simulink library "adrc"  (Simulink 10.0)
settings: Solver=VariableStepAuto  StartTime=0.0  StopTime=10.0  RelTol=1e-3
undefined symbols (not defined in the file): DiscIntNeverNeededParam, Ts
libraries: fl_lib x7, nesl_utility x4, powerlib_meascontrol x1, eeGeneralControl x1
settings Model: Creator=Kamran  LastModifiedBy=Kamran

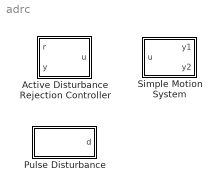
== system adrc ==
  Active Disturbance Rejection Controller : Subsystem  mask(Active Disturbance Rejection Controller){b=1, w=10, n=1, sat=inf}
      mask prompts: b "Input Gain (b)"; w "Bandwidth (w in rad/s)"; n "System Order"; sat "Output Saturation"
      mask help: This simulates a parametrized ADRC controller with minimal number of tuning parameters.
      mask init:
      | A = zeros(n + 1);
      | A(1:end-1, 2:end) = eye(n);
      | 
      | B = zeros(n + 1, 1);
      | B(end-1) = 1;
      | 
      | syms s;
      | 
      | eqn = (s + w) ^ n;
      | c = fliplr(sym2poly(eqn));
      | K = c(1:end-1);
      | 
      | eqn = (s + w) ^ (n + 1);
      | c = sym2poly(eqn);
      | L = c(2:end)';
      mask Display: disp("ADRC")
  Pulse Disturbance : Subsystem  mask{d=2.5, t=0.05, w=2, e=on}
      mask prompts: d "Transport Delay Time"; t "Disturbance Duration"; w "Amplitude"; e "Enabled"
      mask help: Simple pulse disturbance.
      mask Display: disp('Disturbance')
  Simple Motion System : Subsystem  mask{I=2, K=0.2, Taw=1e-3, Ts=1}
      mask prompts: I "Inertia"; K "Damping coefficient"; Taw "Drive Delay"; Ts "Sample Time"
      mask help: Simple motor motion control platform.
      mask Display: disp("Plant")

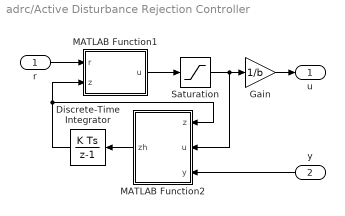
== system adrc/Active Disturbance Rejection Controller ==
  r : Inport
  y : Inport  Port=2
  Discrete-Time Integrator : DiscreteIntegrator  InitialCondition=zeros(1, n + 1)  SampleTime=-1  ICPrevOutput=DiscIntNeverNeededParam  ICPrevScaledInput=DiscIntNeverNeededParam
  Gain : Gain  Gain=1/b
  MATLAB Function1 : MATLAB Function  TreatAsAtomicUnit=on
  MATLAB Function2 : MATLAB Function  TreatAsAtomicUnit=on
  Saturation : Saturate  UpperLimit=sat*b  LowerLimit=-sat*b
  u : Outport  VectorParamsAs1DForOutWhenUnconnected=off
  wires:
  MATLAB Function1/1(u) -> Saturation/1
  r/1 -> MATLAB Function1/1(r)
  Saturation/1 -> Gain/1, MATLAB Function2/2(u)
  y/1 -> MATLAB Function2/3(y)
  Discrete-Time Integrator/1 -> MATLAB Function1/2(z), MATLAB Function2/1(z)
  MATLAB Function2/1(zh) -> Discrete-Time Integrator/1
  Gain/1 -> u/1

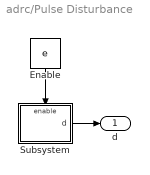
== system adrc/Pulse Disturbance ==
  Enable : Constant  Value=e  SampleTime=Ts
  Subsystem : Subsystem
  d : Outport  VectorParamsAs1DForOutWhenUnconnected=off
  wires:
  Enable/1 -> Subsystem/Enable
  Subsystem/1(d) -> d/1

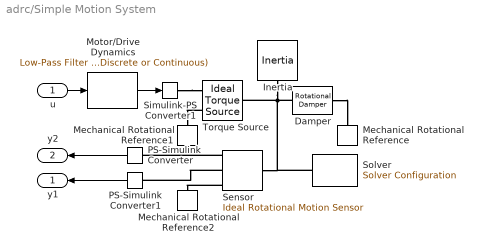
== system adrc/Simple Motion System ==
  u : Inport
  Damper : fl_lib/Mechanical/Rotational Elements/Rotational Damper  D=0.2 N*m/(rad/s)  w_specify=off  w_priority=None  w=0 rad/s  w_nominal_specify=off  w_nominal_unit=rad/s  w_nominal_value=1  t_specify=off  t_priority=None  t=0 N*m  t_nominal_specify=off  t_nominal_unit=N*m  t_nominal_value=1
  Inertia : fl_lib/Mechanical/Rotational Elements/Inertia  inertia=2 kg*m^2  w_specify=off  w_priority=High  w=0 rad/s  w_nominal_specify=off  w_nominal_unit=rad/s  w_nominal_value=1  t_specify=off  t_priority=None  t=0 N*m  t_nominal_specify=off  t_nominal_unit=N*m  t_nominal_value=1
  Mechanical Rotational Reference : fl_lib/Mechanical/Rotational Elements/Mechanical Rotational Reference
  Mechanical Rotational Reference1 : fl_lib/Mechanical/Rotational Elements/Mechanical Rotational Reference
  Mechanical Rotational Reference2 : fl_lib/Mechanical/Rotational Elements/Mechanical Rotational Reference
  Motor/Drive Dynamics : eeGeneralControl/Low-Pass Filter (Discrete or Continuous)  K=1  T=Taw  B=inf  A=-inf  Ts=-1  mask(Low-Pass Filter (Discrete or Continuous)){}
      settings: SourceProductName=Simscape Electrical
      mask Display:
      | % This is a new mask on top of the base mask.
      | % Use "View base mask" link below to see the base mask.
      | plot([0 1 2 3 4], [-1 -1 -2.5 -4 -4])
  PS-Simulink Converter : nesl_utility/PS-Simulink Converter  PhysicalDomain=network_engine_domain  SubClassName=ps_output  LeftPortType=input  RightPortType=output  PseudoPeriodic=off  Frequencies=[]  Unit=rad  AffineConversion=off
  PS-Simulink Converter1 : nesl_utility/PS-Simulink Converter  PhysicalDomain=network_engine_domain  SubClassName=ps_output  LeftPortType=input  RightPortType=output  PseudoPeriodic=off  Frequencies=[]  Unit=rad/s  AffineConversion=off
  Sensor : fl_lib/Mechanical/Mechanical Sensors/Ideal Rotational Motion Sensor  offset=0 rad
  Simulink-PS Converter1 : nesl_utility/Simulink-PS Converter  PhysicalDomain=network_engine_domain  SubClassName=ps_input  LeftPortType=input  RightPortType=output  PseudoPeriodic=off  Frequencies=[]  NoiseDistribution=none  NoiseParameters=[]  Unit=N*m  AffineConversion=off  FilteringAndDerivatives=provide  SimscapeFilterOrder=1  InputFilterTimeConstant=0.001  UdotUserProvided=0
  Solver : nesl_utility/Solver Configuration  PhysicalDomain=network_engine_domain  SubClassName=solver  LeftPortType=input  RightPortType=generic  Tones=[]  Harmonics=[]  SimulateNoise=off  Profile=off  UseLocalSampling=off  EnableSwitchedLinearOptims=on  FrequencyDomain=off  UseCCode=off  RelTol=0.001  AbsTol=1e-06  MinStep=1e-09  ToWorkspace=off  RevertToSquareIcSolve=off  NumHomotopyIterations=100  PhasorMode=off  PhasorModeNumHarmonics=1  DoDC=off  ResidualTolerance=1e-09  UseLocalSolver=on  LocalSolverChoice=NE_BACKWARD_EULER_ADVANCER  LocalSolverSampleTime=Ts  DoFixedCost=off  MaxNonlinIter=3  MaxModeIter=2  LinearAlgebra=auto  EquationFormulation=NE_TIME_EF  DelaysMemoryBudget=1024  AutomaticFiltering=off  FilteringTimeConstant=0.001  PartitionStorageMethod=AS_NEEDED  PartitionMemoryBudget=1024  PartitionMethod=ROBUST
  Torque Source : fl_lib/Mechanical/Mechanical Sources/Ideal Torque Source
  y1 : Outport
  y2 : Outport  Port=2
  wires:
  u/1 -> Motor/Drive Dynamics/1
  PS-Simulink Converter/1 -> y2/1
  Motor/Drive Dynamics/1 -> Simulink-PS Converter1/1
  PS-Simulink Converter1/1 -> y1/1
  connections:
  Inertia/LConn1 -- Torque Source/LConn1 -- Damper/LConn1 -- Solver/RConn1 -- Sensor/LConn1
  Damper/RConn1 -- Mechanical Rotational Reference/LConn1
  Simulink-PS Converter1/RConn1 -- Torque Source/RConn1
  Torque Source/RConn2 -- Mechanical Rotational Reference1/LConn1
  Sensor/RConn3 -- PS-Simulink Converter/LConn1
  Sensor/RConn2 -- PS-Simulink Converter1/LConn1
  Sensor/RConn1 -- Mechanical Rotational Reference2/LConn1

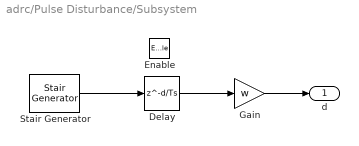
== system adrc/Pulse Disturbance/Subsystem ==
  Enable : EnablePort
  Delay : Delay  DelayLength=d/Ts
  Gain : Gain  Gain=w
  Stair Generator : powerlib_meascontrol/Pulse & Signal Generators/Stair Generator  t=[0, t, 2*t]  e=[1, -1, 0]  Ts=Ts
      settings: SourceProductName=Simscape Electrical
  d : Outport  VectorParamsAs1DForOutWhenUnconnected=off
  wires:
  Stair Generator/1 -> Delay/1
  Gain/1 -> d/1
  Delay/1 -> Gain/1

== matlab function Active Disturbance Rejection Controller/MATLAB Function1 ==
  data: r input double; u output double; z input double; K parameter double
function u = NLSEF(r, z, K)
    u0 = K * (r(1:end-1) - z(1:end-1));
    u = u0 + r(end) - z(end);
end

function x = fe2(e)
    x = zeros(1, 1);
    x(1) = fal(e(1), 1, 0.1);
    x(2) = fal(e(2), 1, 0.001);
end

function x = fe3(e)
    x = zeros(3, 1);
    h = 0.001;
    x(1) = fal(e, 1/1, h);
    x(2) = fal(e, 1/1, h);
    x(3) = fal(e, 1/1, h);
end

function e = fal(x, a, d)
    if abs(x) <= d
        e = x / d ^ (1 - a);
    else
        e = abs(x) ^ a * sign(x);
    end
end

== matlab function Active Disturbance Rejection Controller/MATLAB Function2 ==
  data: z input double; u input double; y input double; A parameter double; zh output double; B parameter double; L parameter double
function zh = ESO(z, u, y, A, B, L)
    zh = A * z + B * u + L * (y - z(1));
end
